simulink model "EMG_no_gaze"  (R2015a)
settings: Solver=ode4  SolverMode=MultiTasking  StartTime=0.0  StopTime=inf  FixedStep=BKIN_STEP_TIME  RelTol=1e-3
StartFcn:
  |  warndlg('Dexterit-E models cannot run under simulation. Please compile your model and run it from within Dexterit-E.');set_param(bdroot,'SimulationCommand','stop')
model workspace (MAT data in the model file):
  BKIN_KINEMATIC_FRAME_SIZE = 400
  BKIN_STEP_TIME = 0.00025
  COLOR = 4
  COL_X = 1
  COL_Y = 2
  E_NO_EVENT = 0
  LOAD_X = 1
  LOAD_Y = 2
  MOVEMENT_DELAY = 3
  PATH_LENGTH = 1
  PATH_PERIOD = 2
  POST_TRIAL_DELAY = 4
  RADIUS = 3
  TRAJECTORY = 1
  TRAJECTORY_TYPE = 2
  TRIAL_END = 3
  TRIAL_MOVEMENT = 2
  TRIAL_RESET = 4
  TRIAL_START = 1
  X_POSITION = 1
  Y_POSITION = 2
  col_x = 1
  col_y = 2
  ANGULAR_THRESHOLD = 5
  GAZE_EXIT = 6
  START_REACHED = 7
  FIXATION_DURATION = 6
  TRACKING_TARGET_ROW = 7
  FEEDBACK_COLOR = 5
  CROSS_LOGICAL_RADIUS = 8
  DETECT_FIXATION = 8
  GAZE_IN_TARGET = 5
  START_STABILIZATION = 9
  HAND_IN_TARGET = 9
  BACKGROUND_LOAD = 10
  PATH_MULTIPLIER = 11
libraries: General x3, Video x2, KINARM_general x1
settings Model: ModifiedComment=chris -- Wed Feb 16 09:18:30 2005 -- Version 1.1384  ModifiedHistory=Feb 16/05 - Add error repeat, add offset ramp  CovHtmlReporting=off  ExtModeArmWhenConnect=off  ExtModeLogAll=off  Creator=Chris Grebeldinger  LastModifiedBy=Brain and Action Lab
settings SolverCC: EnableConcurrentExecution=on  AutoInsertRateTranBlk=on
settings DataIOCC: LimitDataPoints=off  SignalLoggingSaveFormat=ModelDataLogs  SaveOutput=off  SaveTime=off  SignalLoggingName=sigsOut
settings OptimizationCC: BlockReduction=off  BooleanDataType=off  OptimizeBlockIOStorage=off  BufferReuse=off  GlobalBufferReuse=off  ExpressionFolding=off  ExpressionDepthLimit=2147483647  LocalBlockOutputs=off  InitFltsAndDblsToZero=on
settings DebuggingCC: SaveWithParameterizedLinksMsg=none  UnderspecifiedInitializationDetection=Classic  MergeDetectMultiDrivingBlocksExec=none  SignalResolutionControl=TryResolveAllWithWarning  MultiTaskDSMMsg=warning  FcnCallInpInsideContextMsg=EnableAllAsWarning  StateNameClashWarn=warning  StrictBusMsg=ErrorOnBusTreatedAsVector
settings HardwareCC: ProdIntDivRoundTo=Zero  ProdEndianess=LittleEndian  ProdLongLongMode=on  ProdHWDeviceType=Generic->32-bit x86 compatible  TargetHWDeviceType=32-bit Generic
settings SFSimCC: SimCustomSourceCode=#include <stdlib.h>  SimCustomHeaderCode="#include \"stdlib.h\""  SFSimEcho=off  SimParseCustomCode=off
settings RTWCC: SystemTargetFile=slrt.tlc  TemplateMakefile=slrt_default_tmf  Description=Simulink Real-Time  CustomSourceCode="#include \"stdlib.h\""  CodeExecutionProfiling=on
settings CodeAppCC: MaxIdLength=63
settings SimulinkRealTimeCC: TargetFcnLib=ansi_tfl_tmw.mat  GeneratePreprocessorConditionals=Disable all

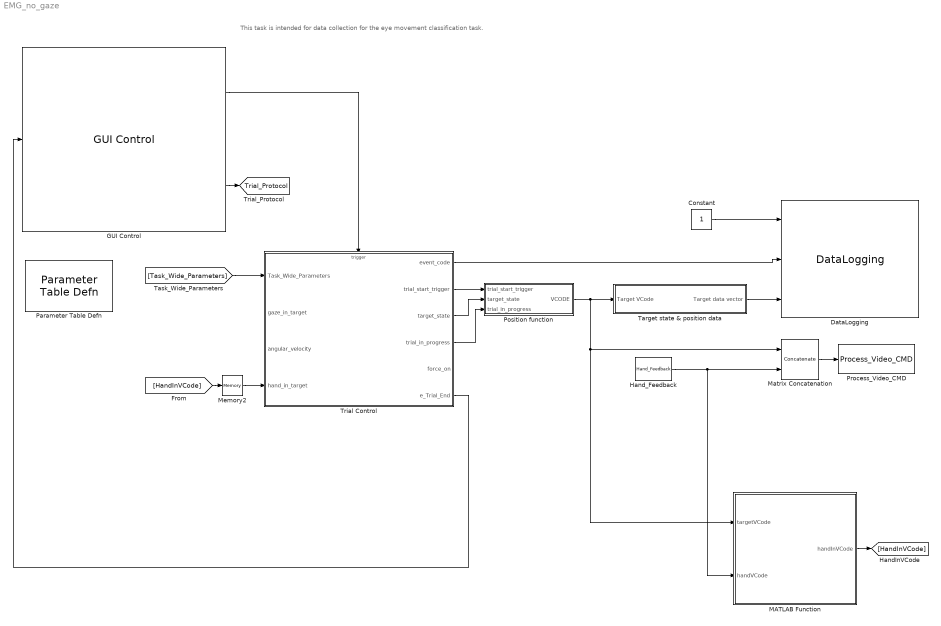
== system EMG_no_gaze ==
  note: This task is intended for data collection for the eye movement classification task.
  Constant : Constant
  DataLogging : General/DataLogging  log_event_codes=on  log_analog_inputs=on  show_time_remaining=off  ecat_include=on
  GUI Control : General/GUI Control  task_version=1.0  show_repeat_trial_flag=off  use_custom_tp=off  target_type_str=Circle  Target_Type=1  XYcols=[1 2]  Vcols=3  Lcols=4  indices_padding=[0 0 0 0;0 0 0 0]  target_table_rows=64  load_table_rows=20  tp_table_rows=100
  Hand_Feedback : KINARM_general/Hand_Feedback  feedback_cntl_src=none
  MATLAB Function : MATLAB Function  TreatAsAtomicUnit=on
  Matrix Concatenation : Concatenate  Mode=Multidimensional array
  Memory2 : Memory
  Parameter Table Defn : General/Parameter Table Defn  ShowInLibBrowser=0
  Position function : Subsystem
  Process_Video_CMD : Video/Process_Video_CMD  video_delay=50
  Target state & position data : Subsystem
  Trial Control : Stateflow chart  TreatAsAtomicUnit=on
  tag scope: Trial_Protocol=global
  wires:
  GUI Control/1 -> Trial Control/Trigger
  Matrix Concatenation/1 -> Process_Video_CMD/1
  Trial Control/6(e_Trial_End) -> GUI Control/1
  Trial Control/2(trial_start_trigger) -> Position function/1(trial_start_trigger)
  [Task_Wide_Parameters] -> Trial Control/1(Task_Wide_Parameters)
  GUI Control/2 -> [Trial_Protocol]
  Hand_Feedback/1 -> MATLAB Function/2(handVCode), Matrix Concatenation/2
  Trial Control/3(target_state) -> Position function/2(target_state)
  Trial Control/4(trial_in_progress) -> Position function/3(trial_in_progress)
  Trial Control/1(event_code) -> DataLogging/2
  Target state & position data/1(Target data vector) -> DataLogging/3
  Position function/1(VCODE) -> Matrix Concatenation/1, MATLAB Function/1(targetVCode), Target state & position data/1(Target VCode)
  Constant/1 -> DataLogging/1
  MATLAB Function/1(handInVCode) -> [HandInVCode]
  Memory2/1 -> Trial Control/4(hand_in_target)
  [HandInVCode] -> Memory2/1

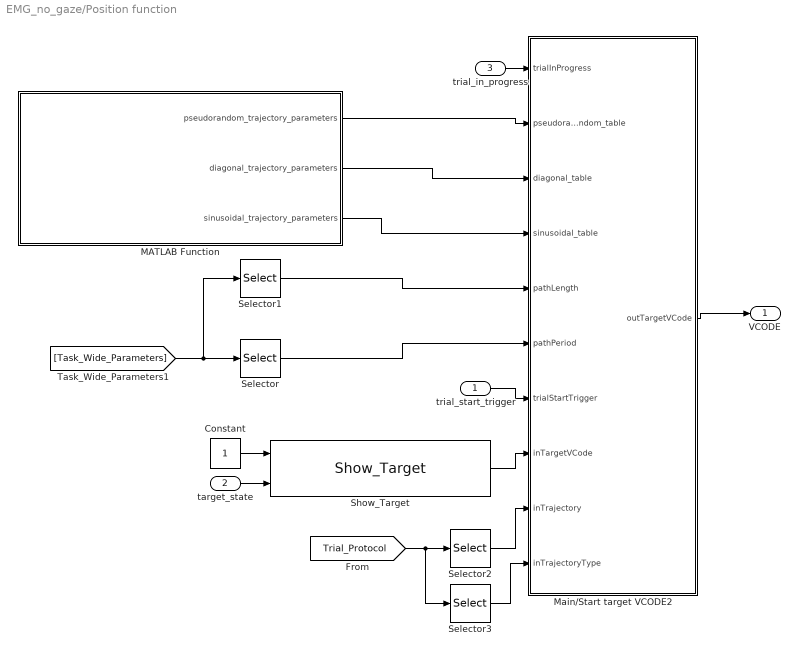
== system EMG_no_gaze/Position function ==
  trial_start_trigger : Inport
  target_state : Inport  Port=2
  trial_in_progress : Inport  Port=3
  Constant : Constant
  MATLAB Function : MATLAB Function  TreatAsAtomicUnit=on
  Main/Start target VCODE2 : MATLAB Function  TreatAsAtomicUnit=on
  Selector : Selector  Indices=PATH_PERIOD
  Selector1 : Selector  Indices=PATH_LENGTH
  Selector2 : Selector  Indices=TRAJECTORY
  Selector3 : Selector  Indices=TRAJECTORY_TYPE
  Show_Target : Video/Show_Target  target_type=Circle  num_states=2  attribcol1=[4 4 0 3]  attribcol2=[5 5 0 3]  attribcol3=[0 0 0 0]  attribcol4=[0 0 0 0]  attribcol5=[0 0 0 0]  stateindices_padding=[0 0 0 0 0 0 0;0 0 0 0 0 0 0;0 0 0 0 0 0 0;0 0 0 0 0 0 0;0 0 0 0 0 0 0]  source=dialog  opacity=100  target_display=Both subject and operator displays  num_col=4
  VCODE : Outport  PortDimensions=[1,70]
  wires:
  Main/Start target VCODE2/1(outTargetVCode) -> VCODE/1
  trial_start_trigger/1 -> Main/Start target VCODE2/7(trialStartTrigger)
  [Task_Wide_Parameters] -> Selector1/1, Selector/1
  Selector/1 -> Main/Start target VCODE2/6(pathPeriod)
  Selector1/1 -> Main/Start target VCODE2/5(pathLength)
  Show_Target/1 -> Main/Start target VCODE2/8(inTargetVCode)
  Constant/1 -> Show_Target/1
  Selector2/1 -> Main/Start target VCODE2/9(inTrajectory)
  [Trial_Protocol] -> Selector3/1, Selector2/1
  target_state/1 -> Show_Target/2
  trial_in_progress/1 -> Main/Start target VCODE2/1(trialInProgress)
  Selector3/1 -> Main/Start target VCODE2/10(inTrajectoryType)
  MATLAB Function/1(pseudorandom_trajectory_parameters) -> Main/Start target VCODE2/2(pseudorandom_table)
  MATLAB Function/2(diagonal_trajectory_parameters) -> Main/Start target VCODE2/3(diagonal_table)
  MATLAB Function/3(sinusoidal_trajectory_parameters) -> Main/Start target VCODE2/4(sinusoidal_table)

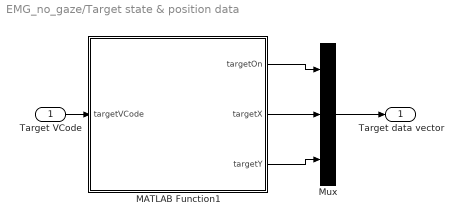
== system EMG_no_gaze/Target state & position data ==
  Target VCode : Inport
  MATLAB Function1 : MATLAB Function  TreatAsAtomicUnit=on
  Mux : Mux  Inputs=3
  Target data vector : Outport
  wires:
  Mux/1 -> Target data vector/1
  Target VCode/1 -> MATLAB Function1/1(targetVCode)
  MATLAB Function1/2(targetX) -> Mux/2
  MATLAB Function1/1(targetOn) -> Mux/1
  MATLAB Function1/3(targetY) -> Mux/3

== matlab function EMG_no_gaze/Target state & position data/MATLAB Function1 ==
  data: targetVCode input; targetOn output; targetX output; targetY output
%This function extracts data to be saved from the target VCode matrix
%(includes both circle & both ellipse targets, not the start target/fixation cross or hand feedback) 
%Returns a vector of doubles.
%VCode order: first circle, first ellipse, second circle, second ellipse
function [targetOn, targetX, targetY] = extractDataChannels(targetVCode)
%#codegen
    onOff = targetVCode(2);
    onOff = typecast(onOff, 'double');
    xPosition = targetVCode(3);
    xPosition = typecast(xPosition, 'double');
    yPosition = targetVCode(4);
    yPosition = typecast(yPosition, 'double');
    
    targetOn = onOff;
    targetX = xPosition;
    targetY = yPosition;
end

== stateflow chart EMG_no_gaze/Trial Control ==
  state Initialiize/
    entry: trial_start_trigger = 0;
    trial_in_progress = 0;
    target_state = 0;
    movement_delay = Task_Wide_Parameters[MOVEMENT_DELAY];//Already in ms
    post_trial_delay = Task_Wide_Parameters[POST_TRIAL_DELAY];//Already in ms
    path_time = Task_Wide_Parameters[PATH_PERIOD] * 1000;//Convert to ms
    event_code = 0;
    trial_start_trigger = 1;
  state MainTrial
    state Start/
      target_state = 1;
      event_code = TRIAL_START;
      state WaitingForHit/
      state HandInStartTarget/
        target_state = 2;
        event_code = START_REACHED;
      (default) -> WaitingForHit
      WaitingForHit -> HandInStartTarget : // has the hand reached the target?
          | [hand_in_target== 1]
      HandInStartTarget -> WaitingForHit [order 2] : // has the hadn left the start target?
          | [hand_in_target == 0]/target_state = 1;
    state SeekingFixation/
      event_code = DETECT_FIXATION;
    state TriggerOn/
      trial_start_trigger = 1;
    state TriggerOff/
      entry: trial_start_trigger = 0;
    state TrialInProgress/
      entry: trial_in_progress = 1;
      event_code = TRIAL_MOVEMENT;
      state HandNotInTarget/
        target_state = 1;
      state HandInTarget/
        event_code = HAND_IN_TARGET;
        target_state = 2;
      (default) -> HandNotInTarget
      HandNotInTarget -> HandInTarget : [hand_in_target == 1]
      HandInTarget -> HandNotInTarget : [hand_in_target == 0]
    state End/
      entry: trial_in_progress = 0;
      event_code = TRIAL_END;
    HandInStartTarget -> SeekingFixation [order 1] : // has the hand remained stable for the specified amount of time?
        | after(Task_Wide_Parameters[START_STABILIZATION],e_clk)
    SeekingFixation -> TriggerOn : after(Task_Wide_Parameters[FIXATION_DURATION], e_clk)
    TriggerOn -> TriggerOff : after(1,e_clk)
    TriggerOff -> TrialInProgress : after(movement_delay, e_clk)
    TrialInProgress -> End : after(path_time, e_clk)
  state Inter_Trial_State/
    // Turn off targets and force, reset the event code, and send the
    //e_Trial_End Stateflow event to indicate that the trial is over.
    entry: target_state = 0;
    event_code = TRIAL_RESET;
    e_Trial_End;
  (default) -> Initialiize
  Initialiize -> Start
  Inter_Trial_State -> Start : // Proceed after post-trial delay
      | after(post_trial_delay, e_clk)
  MainTrial -> Inter_Trial_State : e_ExitTrialNow/
      | // e_ExitTrialNow event occurs if the
      | // Dex pause is pressed by the operator
  End -> Inter_Trial_State
  data: Task_Wide_Parameters input double; event_code output uint16 [0..] =0; trial_start_trigger output boolean; post_trial_delay local double; movement_delay local double; path_time local double; target_state output int8; trial_in_progress output double; gaze_in_target input boolean; angular_velocity input double; hand_in_target input boolean; force_on output boolean
  events: e_clk input RISING_EDGE_EVENT; e_ExitTrialNow input EITHER_EDGE_EVENT; e_Trial_End output EITHER_EDGE_EVENT

== matlab function EMG_no_gaze/Position function/MATLAB Function ==
  data: pseudorandom_trajectory_parameters output; diagonal_trajectory_parameters output; sinusoidal_trajectory_parameters output
function [pseudorandom_trajectory_parameters, diagonal_trajectory_parameters, sinusoidal_trajectory_parameters] = generate_parameter_tables()
    %#codegen
    %Pseudorandom Trajectory Parameter Table Key:
    %Row 1: A1x
    %Row 2: A2x
    %Row 3: Harmonic x
    %Row 4: Phase x (degrees)
    %Row 5: A1y
    %Row 6: A2y
    %Row 7: Harmonic y
    %Row 8: Phase y (degrees)
    pseudorandom_trajectory_parameters = [5,4,4,5,5.1;5,5,5.1,5,5.2;2,2,3,3,2;45,-60,-60,90,-90;5,3,4,3.4,4;5,5,5.2,5,5;3,3,2,2,3;-135,-135,-135,45,22.5];
    
    %Note: This matrix is formulated in (columns, rows) and then transposed
    %Diagonal Trajectory Parameter Table Key:
    %Row 1: Theta (displacement from 0 radians of line)
    %Row 2: Horizontal direction (-1 left, 1 right)
    %Row 3: Vertical direction (-1 down, 1 up)
    diagonal_trajectory_parameters = [15,-1,-1;15,-1,1;15,1,-1;15,1,1;30,-1,-1;30,-1,1;30,1,-1;30,1,1;45,-1,-1;45,-1,1;45,1,-1;45,1,1;60,-1,-1;60,-1,1;60,1,-1;60,1,1;75,-1,-1;75,-1,1;75,1,-1;75,1,1].';
    
    %Note: This matrix is formulated in (columns, rows) and then transposed
    %Sinusoidal Trajectory Parameter Table Key:
    %Row 1: Number of waves (full oscillations) in the path
    %Row 2: Horizontal direction (-1 left, 1 right)
    %Row 3: Vertical direction (-1 down, 1 up)
    sinusoidal_trajectory_parameters = [5,-1,-1;5,-1,1;5,1,-1;5,1,1;10,-1,-1;10,-1,1;10,1,-1;10,1,1;15,-1,-1;15,-1,1;15,1,-1;15,1,1;20,-1,-1;20,-1,1;20,1,-1;20,1,1;25,-1,-1;25,-1,1;25,1,-1;25,1,1].';
end

== matlab function EMG_no_gaze/MATLAB Function ==
  data: targetVCode input; handVCode input; handInVCode output
function handInVCode = handInVCode(targetVCode, handVCode)
% all dimensions in m, rad
% arguments:
% handpos: x,y positions of center of target
% attribcol: columns in target table specifying target attributes.  
% Specific to Target_Type
%	circle:
%	[X0,Y0,r...,rn] where:
%	X0,Y0 : centre of circle
%	r : logical radius of circle (i.e. radius used to determine 'in' or 'out' of target)
%	rn: logical radius of other targets (e.g. 2nd, 3rd) also specified in target row.
%   Up to 4 targets can be specified in a row

handX=handVCode(1,3);
handY=handVCode(1,4);
handRad = handVCode(1,10);
	
targetX = targetVCode(3);
targetY = targetVCode(4);	
deltaX = handX - targetX;
deltaY = handY - targetY;
%circle
radius = targetVCode(10) + handRad;
% simple euclidean distance
distance2 = deltaX.^2 + deltaY.^2;					%distance2 is the square of the distance
handInVCode = (distance2 <= radius.^2);

end

== matlab function EMG_no_gaze/Position function/Main//Start target VCODE2 ==
  data: trialInProgress input; pseudorandom_table input; diagonal_table input; sinusoidal_table input; pathLength input; pathPeriod input; trialStartTrigger input; outTargetVCode output size=[1,70]; inTargetVCode input; inTrajectory input; inTrajectoryType input
function outTargetVCode = generateVCode(trialInProgress, pseudorandom_table, diagonal_table, sinusoidal_table, pathLength, pathPeriod, trialStartTrigger, inTargetVCode, inTrajectory, inTrajectoryType)
%#codegen

    %VCode position values (indices (3) and (4)) are in m, whereas all gain
    %values (e.g. A1x) are in cm and position calculations are completed in
    %cm.
    
    %Trajectory Parameter Table Key:
    %Row 1: A1x
    %Row 2: A2x
    %Row 3: Harmonic x
    %Row 4: Phase x (degrees)
    %Row 5: A1y
    %Row 6: A2y
    %Row 7: Harmonic y
    %Row 8: Phase y (degrees)
    
    %Declare and initialize the variable representing the updated VCode
    newTargetVCode = inTargetVCode;
    
    %Amplitude of sine waves: TODO test values
    a = 3;
    
    %Declare and initialize persistent variables; which define target
    %position, time clock, and trajectory parameters
    persistent targetX targetY targetStartX targetStartY trajectory trajectoryType timeClock parameterTable A1x A2x hx px A1y A2y hy py w numWaves theta rightDirection upDirection;
    if isempty(targetX) || isempty(targetY) || isempty(trajectory) || isempty(trajectoryType) || isempty(timeClock) || isempty(A1x) || isempty(A2x) || isempty(hx) || isempty(px) || isempty(A1y) || isempty(A2y) || isempty(hy) || isempty(py) || isempty(w) || isempty(numWaves) || isempty(theta) || isempty(rightDirection) || isempty(upDirection)
        targetX = -1;
        targetY = -1;
        targetStartX = -1;
        targetStartY = -1;
        timeClock = -1;
        parameterTable = -1;
        A1x = -1;
        A2x = -1;
        hx = -1;
        px = -1;
        A1y = -1;
        A2y = -1;
        hy = -1;
        py = -1;
        w = -1;
        numWaves = -1;
        theta = -1;
        rightDirection = -1;
        upDirection = -1;
        trajectoryType = -1;
        trajectory = -1;
    end
    
    %If the trial start trigger is being fired, generate new velocity & starting target positions for the upcoming trial
    if trialStartTrigger == 1
        trajectory = inTrajectory;%Gives the trajectory number within the trajectory type
        trajectoryType = inTrajectoryType;%Pseudorandom, sinusoidal, diagonal, vertical, or horizontal
        timeClock = 0;
        
        %Set trajectory parameter values for pseudorandom trajectories
        if trajectoryType == 1
            targetX = inTargetVCode(3) * 100;%convert to cm
            targetY = inTargetVCode(4) * 100;%convert to cm
            targetStartX = inTargetVCode(3) * 100;%convert to cm
            targetStartY = inTargetVCode(4) * 100;%convert to cm
            parameterTable = pseudorandom_table;
            A1x = parameterTable(1,trajectory);
            A2x = parameterTable(2,trajectory);
            hx = parameterTable(3,trajectory);
            px = parameterTable(4,trajectory) * (pi / 180);%Convert to radians
            A1y = parameterTable(5,trajectory);
            A2y = parameterTable(6,trajectory);
            hy = parameterTable(7,trajectory);
            py = parameterTable(8,trajectory) * (pi / 180);%Convert to radians
            %Calculate frequency
            w = 1 / pathPeriod;
            
        %Set trajectory parameter values for sinusoidal trajectories
        elseif trajectoryType == 4
            parameterTable = sinusoidal_table;
            numWaves = parameterTable(1,trajectory);
            rightDirection = parameterTable(2,trajectory);
            upDirection = parameterTable(3,trajectory);
            targetX = inTargetVCode(3) * 100 - rightDirection * (pathLength / 2) * 100;%convert to cm
            targetY = inTargetVCode(4) * 100;%convert to cm
            targetStartX = inTargetVCode(3) * 100;%convert to cm
            targetStartY = inTargetVCode(4) * 100;%convert to cm
            
        %Set trajectory parameter values for straight-line trajectories
        else
            parameterTable = diagonal_table;
            theta = parameterTable(1,trajectory);%angle of diagonal line, ignored in horizontal/vertical
            rightDirection = parameterTable(2,trajectory);
            upDirection = parameterTable(3,trajectory);
            if trajectoryType == 2%diagonal
                targetX = inTargetVCode(3) * 100 - rightDirection * (pathLength * cosd(theta) / 2);%convert to cm
                targetY = inTargetVCode(4) * 100 - upDirection * (pathLength * sind(theta) / 2);%convert to cm
                targetStartX = inTargetVCode(3) * 100;%convert to cm
                targetStartY = inTargetVCode(4) * 100;%convert to cm
            elseif trajectoryType == 3%vertical
                targetX = inTargetVCode(3) * 100;%convert to cm
                targetY = inTargetVCode(4) * 100 - upDirection * (pathLength / 2);%convert to cm
                targetStartX = inTargetVCode(3) * 100;%convert to cm
                targetStartY = inTargetVCode(4) * 100;%convert to cm
            else%horizontal
                targetX = inTargetVCode(3) * 100 - rightDirection * (pathLength / 2);%convert to cm
                targetY = inTargetVCode(4) * 100;%convert to cm
                targetStartX = inTargetVCode(3) * 100;%convert to cm
                targetStartY = inTargetVCode(4) * 100;%convert to cm
            end
        end
    end
            
    %If the trial is in progress, update the target position
    if trialInProgress == 1 % The target is displayed
        
        %Set the time value in seconds
        t = timeClock / 4000;%simulation runs at 4 kHz
        
        %Update the position of the target for pseudorandom trajectories
        if trajectoryType == 1
            targetX = targetStartX + (A1x * cos(w * (32/5) * t) + A2x * cos(hx * w * (32/5) * t - px));
            targetY = targetStartY + (A1y * cos(w * (32/5) * t) + A2y * cos(hy * w * (32/5) * t - py));
        elseif trajectoryType == 4 %Update the position of the target for sinusoidal trajectories
            targetX = targetStartX + rightDirection * (t * pathLength / pathPeriod);%TODO change, assumes path length is the horizontal distance (maybe ok? probably not.)
            targetY = targetStartY + upDirection * (t * a * sin(targetX - targetStartX));%TODO factor in number of waves
        elseif trajectoryType == 2 %Update the position of the target for diagonal trajectories
            targetX = targetStartX + rightDirection * (t * pathLength * cosd(theta) / pathPeriod);
            targetY = targetStartY + upDirection * (t * pathLength * sind(theta) / pathPeriod);
        elseif trajectoryType == 3 %Update the position of the target for vertical trajectories
            targetX = targetStartX;
            targetY = targetStartY + upDirection * (t * pathLength/ pathPeriod);
        elseif trajectoryType == 5 %Update the position of the target for horizontal trajectories
            targetX = targetStartX + rightDirection * (t * pathLength/ pathPeriod);
            targetY = targetStartY;
        end
        
        %Update the VCODES to reflect the current x and y positions of the target
        newTargetVCode(3) = targetX * 0.01;%convert to meters
        newTargetVCode(4) = targetY * 0.01;%convert to meters
        
        %Update the clock
        timeClock = timeClock + 1;
    end
    outTime = timeClock;
    outTargetVCode = newTargetVCode;
end
